simulink model "carga_y_twistlocks"  (R2023a)
settings: Solver=VariableStepAuto  StartTime=0.0  StopTime=10.0  RelTol=1e-3
undefined symbols (not defined in the file): b_cx, b_cy, g, H_c, K_cy, M_s
settings Model: Creator=Ferran  LastModifiedBy=Ferran

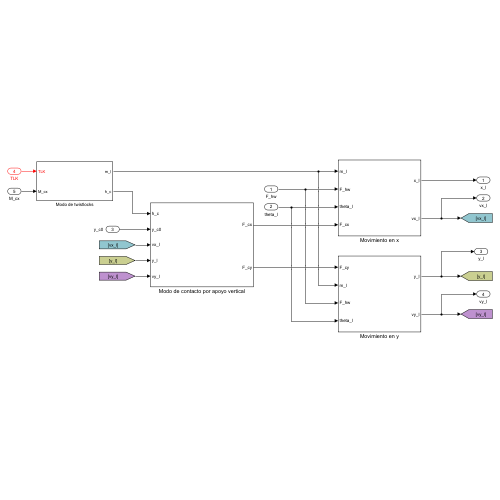
[thumbnail: Simulink's stored preview of the top-level diagram]
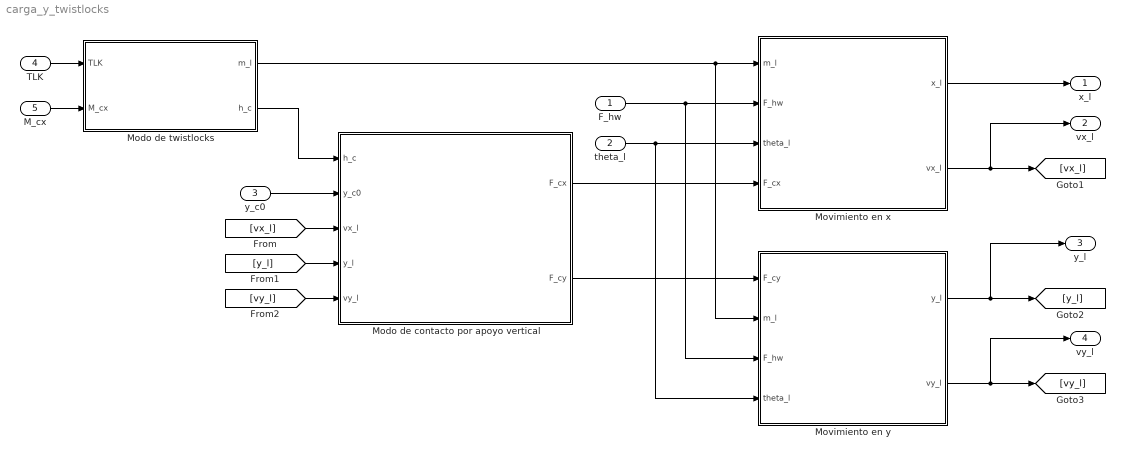
== system carga_y_twistlocks ==
  F_hw : Inport
  theta_l : Inport  Port=2
  y_c0 : Inport  Port=3
  TLK : Inport  Port=4
  M_cx : Inport  Port=5
  Modo de contacto por apoyo vertical : Subsystem
  Modo de twistlocks : Subsystem
  Movimiento en x : Subsystem
  Movimiento en y : Subsystem
  x_l : Outport
  vx_l : Outport  Port=2
  y_l : Outport  Port=3
  vy_l : Outport  Port=4
  wires:
  F_hw/1 -> Movimiento en y/3(F_hw), Movimiento en x/2(F_hw)
  theta_l/1 -> Movimiento en y/4(theta_l), Movimiento en x/3(theta_l)
  Modo de twistlocks/1(m_l) -> Movimiento en x/1(m_l), Movimiento en y/2(m_l)
  Modo de contacto por apoyo vertical/1(F_cx) -> Movimiento en x/4(F_cx)
  Modo de contacto por apoyo vertical/2(F_cy) -> Movimiento en y/1(F_cy)
  Movimiento en x/1(x_l) -> x_l/1
  Movimiento en x/2(vx_l) -> [vx_l], vx_l/1
  Movimiento en y/2(vy_l) -> [vy_l], vy_l/1
  Movimiento en y/1(y_l) -> [y_l], y_l/1
  [vx_l] -> Modo de contacto por apoyo vertical/3(vx_l)
  [y_l] -> Modo de contacto por apoyo vertical/4(y_l)
  [vy_l] -> Modo de contacto por apoyo vertical/5(vy_l)
  y_c0/1 -> Modo de contacto por apoyo vertical/2(y_c0)
  TLK/1 -> Modo de twistlocks/1(TLK)
  M_cx/1 -> Modo de twistlocks/2(M_cx)
  Modo de twistlocks/2(h_c) -> Modo de contacto por apoyo vertical/1(h_c)

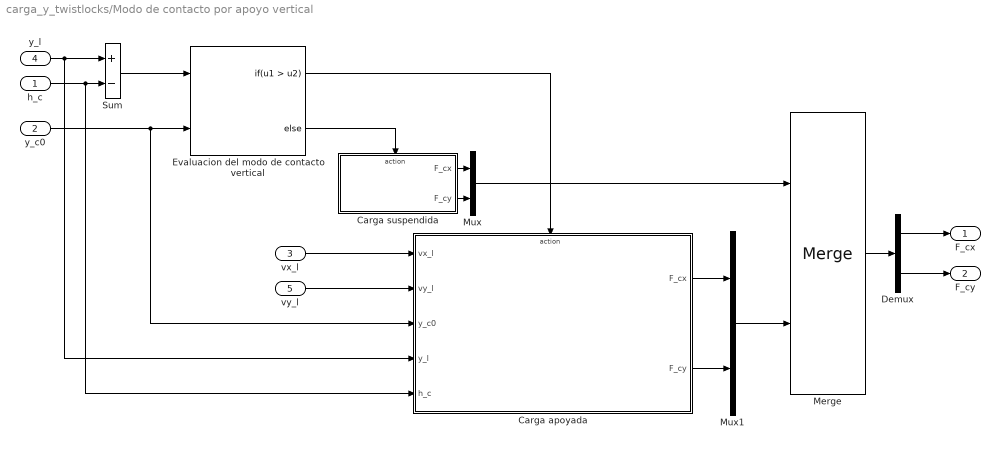
== system carga_y_twistlocks/Modo de contacto por apoyo vertical ==
  h_c : Inport
  y_c0 : Inport  Port=2
  vx_l : Inport  Port=3
  y_l : Inport  Port=4
  vy_l : Inport  Port=5
  Carga apoyada : Subsystem  TreatAsAtomicUnit=on
  Carga suspendida : Subsystem  TreatAsAtomicUnit=on
  Demux : Demux  Outputs=2
  Evaluacion del modo de contacto vertical : If  NumInputs=2  IfExpression=u1 > u2
  Merge : Merge
  Mux : Mux  Inputs=2
  Mux1 : Mux  Inputs=2
  Sum : Sum  Inputs=+-
  F_cx : Outport
  F_cy : Outport  Port=2
  wires:
  Carga apoyada/2(F_cy) -> Mux1/2
  Evaluacion del modo de contacto vertical/1 -> Carga apoyada/Action
  Evaluacion del modo de contacto vertical/2 -> Carga suspendida/Action
  y_c0/1 -> Carga apoyada/3(y_c0), Evaluacion del modo de contacto vertical/2
  vx_l/1 -> Carga apoyada/1(vx_l)
  Sum/1 -> Evaluacion del modo de contacto vertical/1
  y_l/1 -> Carga apoyada/4(y_l), Sum/1
  h_c/1 -> Sum/2, Carga apoyada/5(h_c)
  Carga suspendida/1(F_cx) -> Mux/1
  Carga suspendida/2(F_cy) -> Mux/2
  Mux/1 -> Merge/1
  Carga apoyada/1(F_cx) -> Mux1/1
  Mux1/1 -> Merge/2
  Merge/1 -> Demux/1
  Demux/1 -> F_cx/1
  Demux/2 -> F_cy/1
  vy_l/1 -> Carga apoyada/2(vy_l)

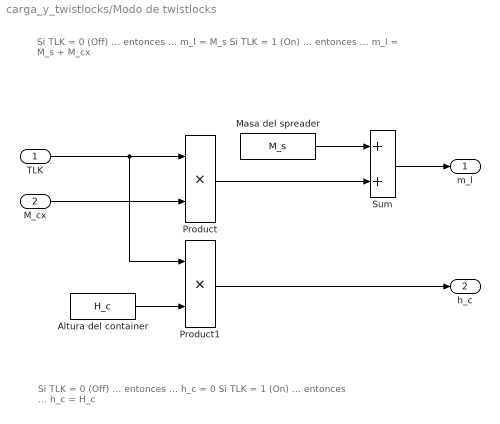
== system carga_y_twistlocks/Modo de twistlocks ==
  note: Si TLK = 0 (Off) ... entonces ... h_c = 0
      | Si TLK = 1 (On) ... entonces ... h_c = H_c
  note: Si TLK = 0 (Off) ... entonces ... m_l = M_s
      | Si TLK = 1 (On) ... entonces ... m_l = M_s + M_cx
  TLK : Inport
  M_cx : Inport  Port=2
  Altura del container : Constant  Value=H_c
  Masa del spreader : Constant  Value=M_s
  Product : Product
  Product1 : Product
  Sum : Sum
  m_l : Outport
  h_c : Outport  Port=2
  wires:
  M_cx/1 -> Product/2
  Sum/1 -> m_l/1
  TLK/1 -> Product/1, Product1/1
  Masa del spreader/1 -> Sum/1
  Product/1 -> Sum/2
  Altura del container/1 -> Product1/2
  Product1/1 -> h_c/1

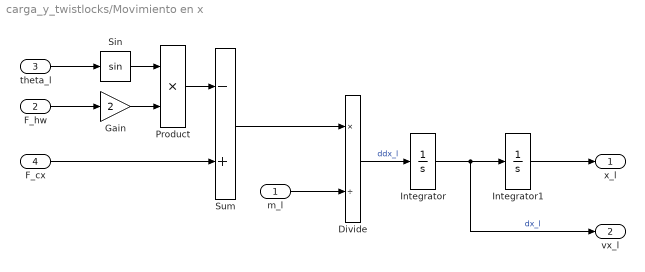
== system carga_y_twistlocks/Movimiento en x ==
  m_l : Inport
  F_hw : Inport  Port=2
  theta_l : Inport  Port=3
  F_cx : Inport  Port=4
  Divide : Product  Inputs=*/
  Gain : Gain  Gain=2
  Integrator : Integrator
  Integrator1 : Integrator
  Product : Product
  Sin : Trigonometry
  Sum : Sum  Inputs=-+
  x_l : Outport
  vx_l : Outport  Port=2
  wires:
  Integrator1/1 -> x_l/1
  Product/1 -> Sum/1
  Sum/1 -> Divide/1
  m_l/1 -> Divide/2
  Integrator/1 -> vx_l/1, Integrator1/1  "dx_l"
  Sin/1 -> Product/1
  theta_l/1 -> Sin/1
  F_cx/1 -> Sum/2
  Divide/1 -> Integrator/1  "ddx_l"
  F_hw/1 -> Gain/1
  Gain/1 -> Product/2

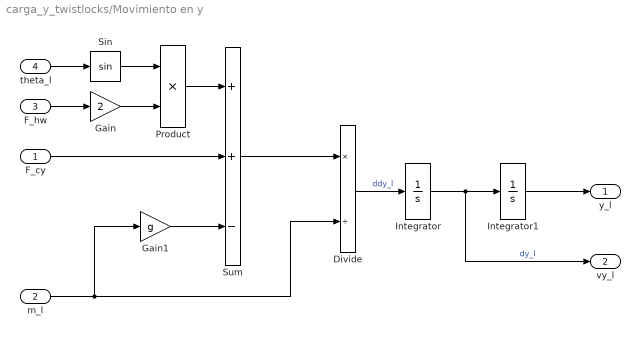
== system carga_y_twistlocks/Movimiento en y ==
  F_cy : Inport
  m_l : Inport  Port=2
  F_hw : Inport  Port=3
  theta_l : Inport  Port=4
  Divide : Product  Inputs=*/
  Gain : Gain  Gain=2
  Gain1 : Gain  Gain=g
  Integrator : Integrator
  Integrator1 : Integrator
  Product : Product
  Sin : Trigonometry
  Sum : Sum  Inputs=++-
  y_l : Outport
  vy_l : Outport  Port=2
  wires:
  Integrator1/1 -> y_l/1
  Product/1 -> Sum/1
  Sum/1 -> Divide/1
  m_l/1 -> Divide/2, Gain1/1
  Integrator/1 -> vy_l/1, Integrator1/1  "dy_l"
  Sin/1 -> Product/1
  theta_l/1 -> Sin/1
  F_cy/1 -> Sum/2
  Divide/1 -> Integrator/1  "ddy_l"
  F_hw/1 -> Gain/1
  Gain/1 -> Product/2
  Gain1/1 -> Sum/3

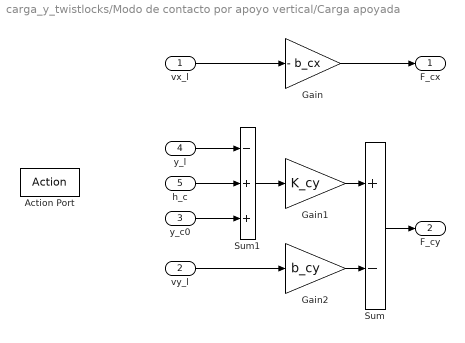
== system carga_y_twistlocks/Modo de contacto por apoyo vertical/Carga apoyada ==
  vx_l : Inport
  vy_l : Inport  Port=2
  y_c0 : Inport  Port=3
  y_l : Inport  Port=4
  h_c : Inport  Port=5
  Action Port : ActionPort  ActionPortLabel=if(u1 > u2)
  Gain : Gain  Gain=- b_cx
  Gain1 : Gain  Gain=K_cy
  Gain2 : Gain  Gain=b_cy
  Sum : Sum  Inputs=+-
  Sum1 : Sum  Inputs=-++
  F_cx : Outport
  F_cy : Outport  Port=2
  wires:
  vx_l/1 -> Gain/1
  Gain/1 -> F_cx/1
  Gain1/1 -> Sum/1
  Sum/1 -> F_cy/1
  Gain2/1 -> Sum/2
  vy_l/1 -> Gain2/1
  Sum1/1 -> Gain1/1
  y_l/1 -> Sum1/1
  h_c/1 -> Sum1/2
  y_c0/1 -> Sum1/3

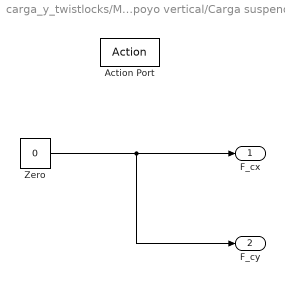
== system carga_y_twistlocks/Modo de contacto por apoyo vertical/Carga suspendida ==
  Action Port : ActionPort  ActionPortLabel=else
  Zero : Constant  Value=0  OutDataTypeStr=Inherit: Inherit via back propagation
  F_cx : Outport
  F_cy : Outport  Port=2
  wires:
  Zero/1 -> F_cx/1, F_cy/1
